simulink model "Wiper_Model"  (R2022b)
settings: Solver=FixedStepAuto  StartTime=0.0  StopTime=10.0  FixedStep=0.01  RelTol=1e-3
libraries: simulink x1
settings Model: Creator=suha274823  LastModifiedBy=suha274823
settings ConfigComp: CovEnable=on  RecordCoverage=on  CovSaveSingleToWorkspaceVar=on  CovModelRefEnable=on

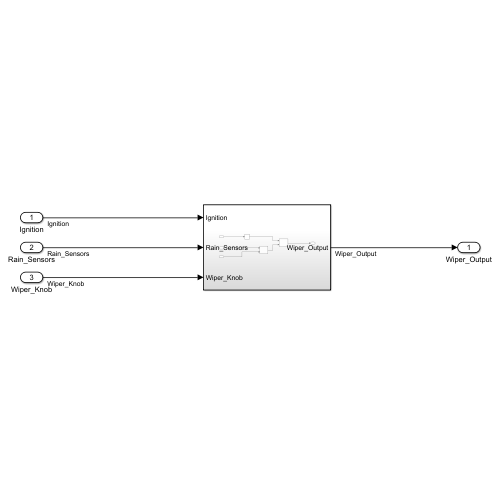
[thumbnail: Simulink's stored preview of the top-level diagram]
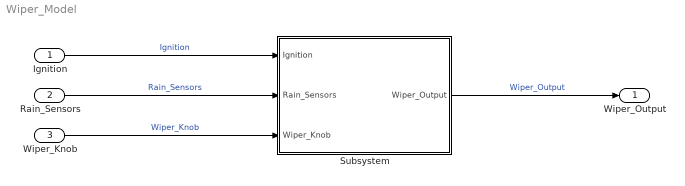
== system Wiper_Model ==
  Ignition : Inport
  Rain_Sensors : Inport  Port=2
  Wiper_Knob : Inport  Port=3
  Subsystem : Subsystem
  Wiper_Output : Outport
  wires:
  Ignition/1 -> Subsystem/1(Ignition)  "Ignition"
  Rain_Sensors/1 -> Subsystem/2(Rain_Sensors)  "Rain_Sensors"
  Wiper_Knob/1 -> Subsystem/3(Wiper_Knob)  "Wiper_Knob"
  Subsystem/1(Wiper_Output) -> Wiper_Output/1  "Wiper_Output"

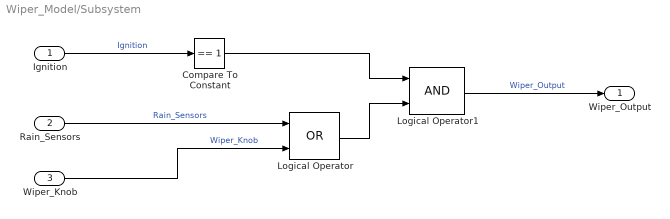
== system Wiper_Model/Subsystem ==
  Ignition : Inport
  Rain_Sensors : Inport  Port=2
  Wiper_Knob : Inport  Port=3
  Compare To Constant : simulink/Logic and Bit Operations/Compare To Constant  relop===  const=1  OutDataTypeStr=boolean
  Logical Operator : Logic  Operator=OR  AllPortsSameDT=off  OutDataTypeStr=boolean
  Logical Operator1 : Logic  AllPortsSameDT=off  OutDataTypeStr=boolean
  Wiper_Output : Outport
  wires:
  Logical Operator/1 -> Logical Operator1/2
  Logical Operator1/1 -> Wiper_Output/1  "Wiper_Output"
  Compare To Constant/1 -> Logical Operator1/1
  Rain_Sensors/1 -> Logical Operator/1  "Rain_Sensors"
  Wiper_Knob/1 -> Logical Operator/2  "Wiper_Knob"
  Ignition/1 -> Compare To Constant/1  "Ignition"
